simulink model "DrivingSimVR"  (Simulink 7.8)
settings: Solver=ode3  StartTime=0.0  StopTime=1000  FixedStep=0.05  RelTol=1e-3
PostLoadFcn:
  | load position
undefined symbols (not defined in the file or in its folder): serial
libraries: Conv_Lib x22, instrumentlib x2, vrlib x1
settings Model: Creator=CYJ  LastModifiedBy=rmchapin
settings DebuggingCC: FcnCallInpInsideContextMsg=Use local settings  StrictBusMsg=Warning

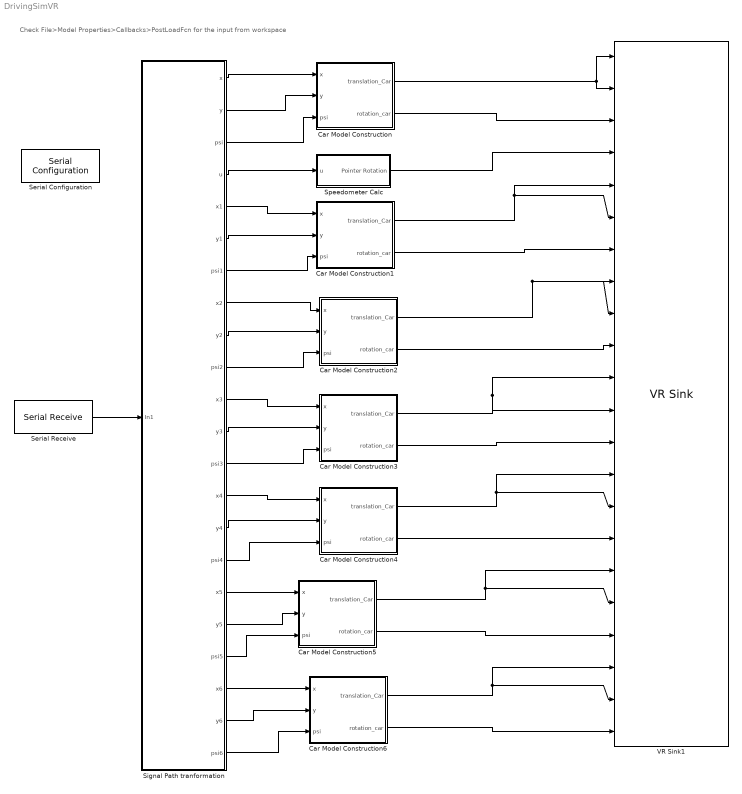
== system DrivingSimVR ==
  note: Check File>Model Properties>Callbacks>PostLoadFcn for the input from workspace
  Car Model Construction : Subsystem
  Car Model Construction1 : Subsystem
  Car Model Construction2 : Subsystem
  Car Model Construction3 : Subsystem
  Car Model Construction4 : Subsystem
  Car Model Construction5 : Subsystem
  Car Model Construction6 : Subsystem
  Serial Configuration : instrumentlib/Serial Configuration  Priority=-200000  ComPortMenu=COM1  ComPort=COM1  ObjConstructor=serial('COM1');  BaudRate=115200  DataBits=8  Parity=none  StopBits=1  FlowControl=none  Timeout=10  ByteOrder=BigEndian
  Serial Receive : instrumentlib/Serial Receive  ComPortMenu=COM1  ComPort=COM1  ObjConstructor=serial('COM1');  Header=s  Terminator=e  DataSize="[88   1]"  DataType=uint8  EnableBlockingMode=on  ActionDataUnavailable=Error  CustomValue=0  SampleTime=0.05
  Signal Path tranformation : Subsystem
  Speedometer Calc : Subsystem
  VR Sink1 : vrlib/VR Sink  SampleTime=0.05  ViewEnable=on  RemoteChange=off  RemoteView=off  FieldsWritten=Vehicle1.translation.3.1.1.double#Object1.translation.3.1.1.double#Car_Lotus1.rotation.4.1.1.double#Pointer.rotation.4.1.1.double#Vehicle2.translation.3.1.1.double#Object2.translation.3.1.1.double#Car_Lotus2.rotation.4.1.1.double#Vehicle3.translation.3.1.1.double#Object3.translation.3.1.1.double#Car_Lotus3.rotation.4.1.1.double#Vehicle4.translation.3.1.1.double#Object4.translation.3.1.1.double#Car_Lotus4.rotation.4.1.1.double#Vehicle5.translation.3.1.1.double#Object5.translation.3.1.1.double#Car_Lotus5.rotation.4.1.1.double#Vehicle6.translation.3.1.1.double#Object6.translation.3.1.1.double#Car_Lotus6.rotation.4.1.1.double#Vehicle7.translation.3.1.1.double#Object7.translation.3.1.1.double#Car_Lotus7.rotation.4.1.1.double  WorldFileName=path-11052012.wrl  AutoView=on  VideoDimensions=[]  AllowVariableSize=off
  wires:
  Serial Receive/1 -> Signal Path tranformation/1(In1)
  Signal Path tranformation/1(x) -> Car Model Construction/1(x)
  Signal Path tranformation/2(y) -> Car Model Construction/2(y)
  Signal Path tranformation/3(psi) -> Car Model Construction/3(psi)
  Signal Path tranformation/5(x1) -> Car Model Construction1/1(x)
  Signal Path tranformation/6(y1) -> Car Model Construction1/2(y)
  Signal Path tranformation/7(psi1) -> Car Model Construction1/3(psi)
  Signal Path tranformation/8(x2) -> Car Model Construction2/1(x)
  Signal Path tranformation/9(y2) -> Car Model Construction2/2(y)
  Signal Path tranformation/10(psi2) -> Car Model Construction2/3(psi)
  Signal Path tranformation/11(x3) -> Car Model Construction3/1(x)
  Signal Path tranformation/12(y3) -> Car Model Construction3/2(y)
  Signal Path tranformation/13(psi3) -> Car Model Construction3/3(psi)
  Signal Path tranformation/14(x4) -> Car Model Construction4/1(x)
  Signal Path tranformation/15(y4) -> Car Model Construction4/2(y)
  Signal Path tranformation/16(psi4) -> Car Model Construction4/3(psi)
  Signal Path tranformation/17(x5) -> Car Model Construction5/1(x)
  Signal Path tranformation/18(y5) -> Car Model Construction5/2(y)
  Signal Path tranformation/19(psi5) -> Car Model Construction5/3(psi)
  Signal Path tranformation/4(u) -> Speedometer Calc/1(u)
  Car Model Construction/1(translation_Car) -> VR Sink1/1, VR Sink1/2
  Car Model Construction1/1(translation_Car) -> VR Sink1/5, VR Sink1/6
  Car Model Construction/2(rotation_car) -> VR Sink1/3
  Speedometer Calc/1(Pointer Rotation) -> VR Sink1/4
  Car Model Construction1/2(rotation_car) -> VR Sink1/7
  Car Model Construction2/1(translation_Car) -> VR Sink1/8, VR Sink1/9
  Car Model Construction2/2(rotation_car) -> VR Sink1/10
  Car Model Construction3/1(translation_Car) -> VR Sink1/11, VR Sink1/12
  Car Model Construction3/2(rotation_car) -> VR Sink1/13
  Car Model Construction4/1(translation_Car) -> VR Sink1/14, VR Sink1/15
  Car Model Construction4/2(rotation_car) -> VR Sink1/16
  Car Model Construction5/1(translation_Car) -> VR Sink1/17, VR Sink1/18
  Car Model Construction5/2(rotation_car) -> VR Sink1/19
  Signal Path tranformation/20(x6) -> Car Model Construction6/1(x)
  Signal Path tranformation/21(y6) -> Car Model Construction6/2(y)
  Signal Path tranformation/22(psi6) -> Car Model Construction6/3(psi)
  Car Model Construction6/1(translation_Car) -> VR Sink1/20, VR Sink1/21
  Car Model Construction6/2(rotation_car) -> VR Sink1/22

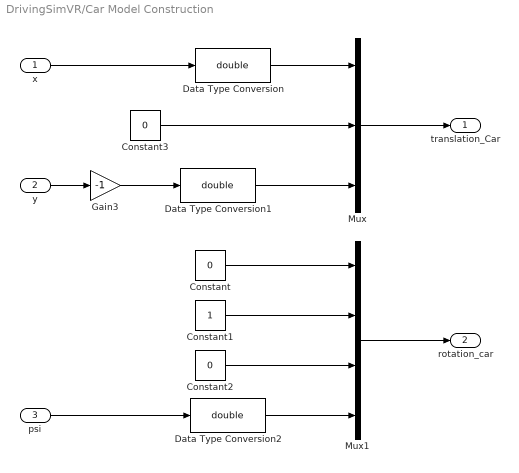
== system DrivingSimVR/Car Model Construction ==
  x : Inport
  y : Inport  Port=2
  psi : Inport  Port=3
  Constant : Constant  Value=0
  Constant1 : Constant
  Constant2 : Constant  Value=0
  Constant3 : Constant  Value=0
  Data Type Conversion : DataTypeConversion  OutDataTypeStr=double
  Data Type Conversion1 : DataTypeConversion  OutDataTypeStr=double
  Data Type Conversion2 : DataTypeConversion  OutDataTypeStr=double
  Gain3 : Gain  Gain=-1
  Mux : Mux  Inputs=3
  Mux1 : Mux
  translation_Car : Outport
  rotation_car : Outport  Port=2
  wires:
  Constant/1 -> Mux1/1
  Constant1/1 -> Mux1/2
  Constant2/1 -> Mux1/3
  Data Type Conversion2/1 -> Mux1/4
  y/1 -> Gain3/1
  psi/1 -> Data Type Conversion2/1
  Constant3/1 -> Mux/2
  Gain3/1 -> Data Type Conversion1/1
  x/1 -> Data Type Conversion/1
  Data Type Conversion1/1 -> Mux/3
  Data Type Conversion/1 -> Mux/1
  Mux/1 -> translation_Car/1
  Mux1/1 -> rotation_car/1

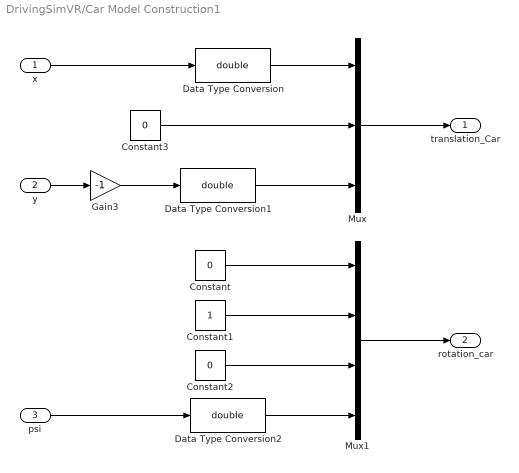
== system DrivingSimVR/Car Model Construction1 ==
  x : Inport
  y : Inport  Port=2
  psi : Inport  Port=3
  Constant : Constant  Value=0
  Constant1 : Constant
  Constant2 : Constant  Value=0
  Constant3 : Constant  Value=0
  Data Type Conversion : DataTypeConversion  OutDataTypeStr=double
  Data Type Conversion1 : DataTypeConversion  OutDataTypeStr=double
  Data Type Conversion2 : DataTypeConversion  OutDataTypeStr=double
  Gain3 : Gain  Gain=-1
  Mux : Mux  Inputs=3
  Mux1 : Mux
  translation_Car : Outport
  rotation_car : Outport  Port=2
  wires:
  Constant/1 -> Mux1/1
  Constant1/1 -> Mux1/2
  Constant2/1 -> Mux1/3
  Data Type Conversion2/1 -> Mux1/4
  y/1 -> Gain3/1
  psi/1 -> Data Type Conversion2/1
  Constant3/1 -> Mux/2
  Gain3/1 -> Data Type Conversion1/1
  x/1 -> Data Type Conversion/1
  Data Type Conversion1/1 -> Mux/3
  Data Type Conversion/1 -> Mux/1
  Mux/1 -> translation_Car/1
  Mux1/1 -> rotation_car/1

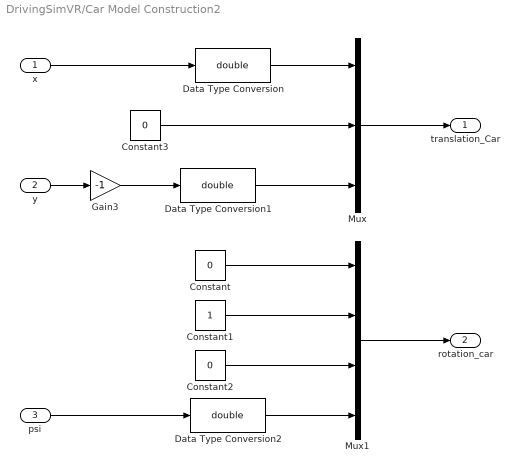
== system DrivingSimVR/Car Model Construction2 ==
  x : Inport
  y : Inport  Port=2
  psi : Inport  Port=3
  Constant : Constant  Value=0
  Constant1 : Constant
  Constant2 : Constant  Value=0
  Constant3 : Constant  Value=0
  Data Type Conversion : DataTypeConversion  OutDataTypeStr=double
  Data Type Conversion1 : DataTypeConversion  OutDataTypeStr=double
  Data Type Conversion2 : DataTypeConversion  OutDataTypeStr=double
  Gain3 : Gain  Gain=-1
  Mux : Mux  Inputs=3
  Mux1 : Mux
  translation_Car : Outport
  rotation_car : Outport  Port=2
  wires:
  Constant/1 -> Mux1/1
  Constant1/1 -> Mux1/2
  Constant2/1 -> Mux1/3
  Data Type Conversion2/1 -> Mux1/4
  y/1 -> Gain3/1
  psi/1 -> Data Type Conversion2/1
  Constant3/1 -> Mux/2
  Gain3/1 -> Data Type Conversion1/1
  x/1 -> Data Type Conversion/1
  Data Type Conversion1/1 -> Mux/3
  Data Type Conversion/1 -> Mux/1
  Mux/1 -> translation_Car/1
  Mux1/1 -> rotation_car/1

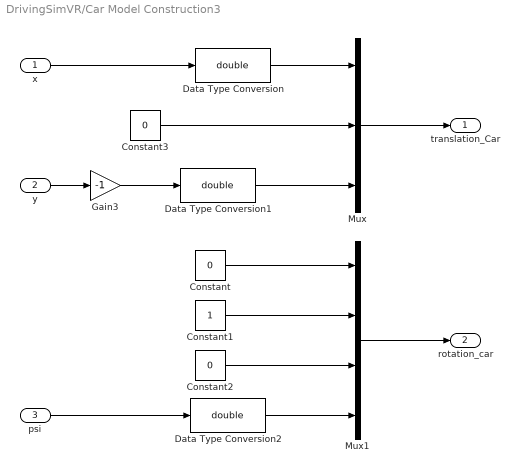
== system DrivingSimVR/Car Model Construction3 ==
  x : Inport
  y : Inport  Port=2
  psi : Inport  Port=3
  Constant : Constant  Value=0
  Constant1 : Constant
  Constant2 : Constant  Value=0
  Constant3 : Constant  Value=0
  Data Type Conversion : DataTypeConversion  OutDataTypeStr=double
  Data Type Conversion1 : DataTypeConversion  OutDataTypeStr=double
  Data Type Conversion2 : DataTypeConversion  OutDataTypeStr=double
  Gain3 : Gain  Gain=-1
  Mux : Mux  Inputs=3
  Mux1 : Mux
  translation_Car : Outport
  rotation_car : Outport  Port=2
  wires:
  Constant/1 -> Mux1/1
  Constant1/1 -> Mux1/2
  Constant2/1 -> Mux1/3
  Data Type Conversion2/1 -> Mux1/4
  y/1 -> Gain3/1
  psi/1 -> Data Type Conversion2/1
  Constant3/1 -> Mux/2
  Gain3/1 -> Data Type Conversion1/1
  x/1 -> Data Type Conversion/1
  Data Type Conversion1/1 -> Mux/3
  Data Type Conversion/1 -> Mux/1
  Mux/1 -> translation_Car/1
  Mux1/1 -> rotation_car/1

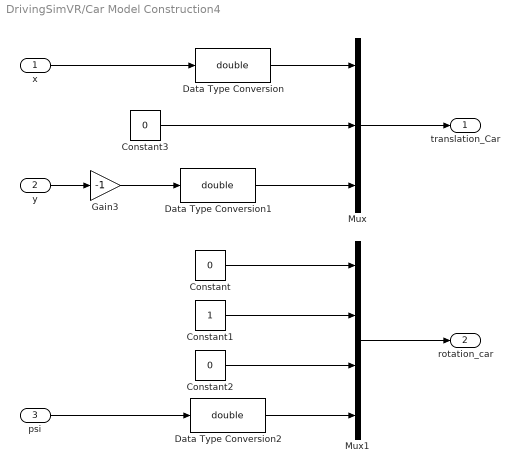
== system DrivingSimVR/Car Model Construction4 ==
  x : Inport
  y : Inport  Port=2
  psi : Inport  Port=3
  Constant : Constant  Value=0
  Constant1 : Constant
  Constant2 : Constant  Value=0
  Constant3 : Constant  Value=0
  Data Type Conversion : DataTypeConversion  OutDataTypeStr=double
  Data Type Conversion1 : DataTypeConversion  OutDataTypeStr=double
  Data Type Conversion2 : DataTypeConversion  OutDataTypeStr=double
  Gain3 : Gain  Gain=-1
  Mux : Mux  Inputs=3
  Mux1 : Mux
  translation_Car : Outport
  rotation_car : Outport  Port=2
  wires:
  Constant/1 -> Mux1/1
  Constant1/1 -> Mux1/2
  Constant2/1 -> Mux1/3
  Data Type Conversion2/1 -> Mux1/4
  y/1 -> Gain3/1
  psi/1 -> Data Type Conversion2/1
  Constant3/1 -> Mux/2
  Gain3/1 -> Data Type Conversion1/1
  x/1 -> Data Type Conversion/1
  Data Type Conversion1/1 -> Mux/3
  Data Type Conversion/1 -> Mux/1
  Mux/1 -> translation_Car/1
  Mux1/1 -> rotation_car/1

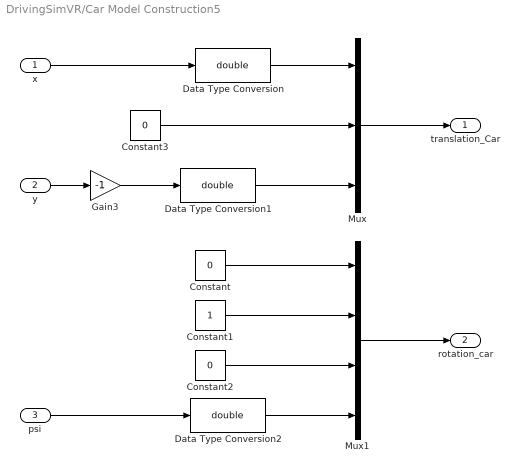
== system DrivingSimVR/Car Model Construction5 ==
  x : Inport
  y : Inport  Port=2
  psi : Inport  Port=3
  Constant : Constant  Value=0
  Constant1 : Constant
  Constant2 : Constant  Value=0
  Constant3 : Constant  Value=0
  Data Type Conversion : DataTypeConversion  OutDataTypeStr=double
  Data Type Conversion1 : DataTypeConversion  OutDataTypeStr=double
  Data Type Conversion2 : DataTypeConversion  OutDataTypeStr=double
  Gain3 : Gain  Gain=-1
  Mux : Mux  Inputs=3
  Mux1 : Mux
  translation_Car : Outport
  rotation_car : Outport  Port=2
  wires:
  Constant/1 -> Mux1/1
  Constant1/1 -> Mux1/2
  Constant2/1 -> Mux1/3
  Data Type Conversion2/1 -> Mux1/4
  y/1 -> Gain3/1
  psi/1 -> Data Type Conversion2/1
  Constant3/1 -> Mux/2
  Gain3/1 -> Data Type Conversion1/1
  x/1 -> Data Type Conversion/1
  Data Type Conversion1/1 -> Mux/3
  Data Type Conversion/1 -> Mux/1
  Mux/1 -> translation_Car/1
  Mux1/1 -> rotation_car/1

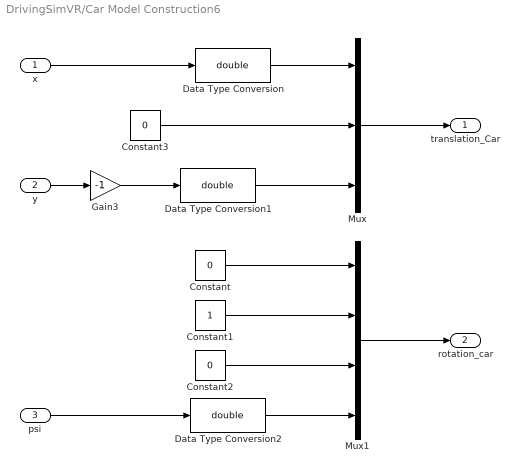
== system DrivingSimVR/Car Model Construction6 ==
  x : Inport
  y : Inport  Port=2
  psi : Inport  Port=3
  Constant : Constant  Value=0
  Constant1 : Constant
  Constant2 : Constant  Value=0
  Constant3 : Constant  Value=0
  Data Type Conversion : DataTypeConversion  OutDataTypeStr=double
  Data Type Conversion1 : DataTypeConversion  OutDataTypeStr=double
  Data Type Conversion2 : DataTypeConversion  OutDataTypeStr=double
  Gain3 : Gain  Gain=-1
  Mux : Mux  Inputs=3
  Mux1 : Mux
  translation_Car : Outport
  rotation_car : Outport  Port=2
  wires:
  Constant/1 -> Mux1/1
  Constant1/1 -> Mux1/2
  Constant2/1 -> Mux1/3
  Data Type Conversion2/1 -> Mux1/4
  y/1 -> Gain3/1
  psi/1 -> Data Type Conversion2/1
  Constant3/1 -> Mux/2
  Gain3/1 -> Data Type Conversion1/1
  x/1 -> Data Type Conversion/1
  Data Type Conversion1/1 -> Mux/3
  Data Type Conversion/1 -> Mux/1
  Mux/1 -> translation_Car/1
  Mux1/1 -> rotation_car/1

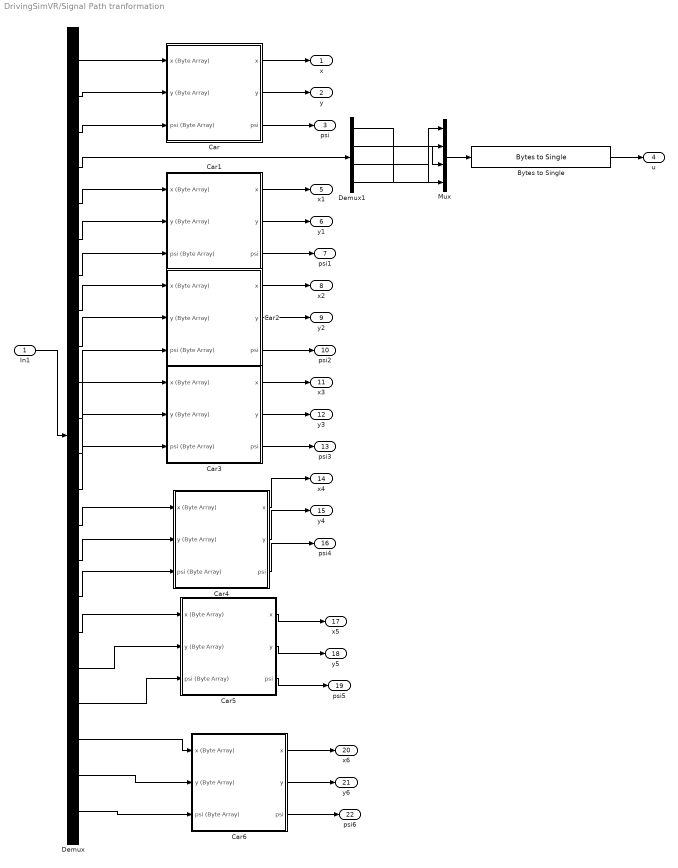
== system DrivingSimVR/Signal Path tranformation ==
  In1 : Inport
  Bytes to Single : Conv_Lib/Bytes to Single
  Car : Subsystem
  Car1 : Subsystem
  Car2 : Subsystem
  Car3 : Subsystem
  Car4 : Subsystem
  Car5 : Subsystem
  Car6 : Subsystem
  Demux : Demux  Outputs=22
  Demux1 : Demux
  Mux : Mux
  x : Outport
  y : Outport  Port=2
  psi : Outport  Port=3
  u : Outport  Port=4
  x1 : Outport  Port=5
  y1 : Outport  Port=6
  psi1 : Outport  Port=7
  x2 : Outport  Port=8
  y2 : Outport  Port=9
  psi2 : Outport  Port=10
  x3 : Outport  Port=11
  y3 : Outport  Port=12
  psi3 : Outport  Port=13
  x4 : Outport  Port=14
  y4 : Outport  Port=15
  psi4 : Outport  Port=16
  x5 : Outport  Port=17
  y5 : Outport  Port=18
  psi5 : Outport  Port=19
  x6 : Outport  Port=20
  y6 : Outport  Port=21
  psi6 : Outport  Port=22
  wires:
  In1/1 -> Demux/1
  Car/1(x) -> x/1
  Car/2(y) -> y/1
  Car/3(psi) -> psi/1
  Demux/1 -> Car/1(x (Byte Array))
  Demux/2 -> Car/2(y (Byte Array))
  Demux/3 -> Car/3(psi (Byte Array))
  Bytes to Single/1 -> u/1
  Car1/1(x) -> x1/1
  Car1/2(y) -> y1/1
  Car1/3(psi) -> psi1/1
  Car2/1(x) -> x2/1
  Car2/2(y) -> y2/1
  Car2/3(psi) -> psi2/1
  Car3/1(x) -> x3/1
  Car3/2(y) -> y3/1
  Car3/3(psi) -> psi3/1
  Car4/1(x) -> x4/1
  Car4/2(y) -> y4/1
  Car4/3(psi) -> psi4/1
  Car5/1(x) -> x5/1
  Car5/2(y) -> y5/1
  Car5/3(psi) -> psi5/1
  Demux/5 -> Car1/1(x (Byte Array))
  Demux/6 -> Car1/2(y (Byte Array))
  Demux/7 -> Car1/3(psi (Byte Array))
  Demux/8 -> Car2/1(x (Byte Array))
  Demux/9 -> Car2/2(y (Byte Array))
  Demux/10 -> Car2/3(psi (Byte Array))
  Demux/11 -> Car3/1(x (Byte Array))
  Demux/12 -> Car3/2(y (Byte Array))
  Demux/13 -> Car3/3(psi (Byte Array))
  Demux/14 -> Car4/1(x (Byte Array))
  Demux/15 -> Car4/2(y (Byte Array))
  Demux/16 -> Car4/3(psi (Byte Array))
  Mux/1 -> Bytes to Single/1
  Demux1/1 -> Mux/4
  Demux1/2 -> Mux/3
  Demux1/3 -> Mux/2
  Demux1/4 -> Mux/1
  Demux/4 -> Demux1/1
  Car6/1(x) -> x6/1
  Car6/2(y) -> y6/1
  Car6/3(psi) -> psi6/1
  Demux/17 -> Car5/1(x (Byte Array))
  Demux/18 -> Car5/2(y (Byte Array))
  Demux/19 -> Car5/3(psi (Byte Array))
  Demux/20 -> Car6/1(x (Byte Array))
  Demux/21 -> Car6/2(y (Byte Array))
  Demux/22 -> Car6/3(psi (Byte Array))

== system DrivingSimVR/Speedometer Calc ==
  u : Inport
  Constant : Constant  Value=0
  Constant1 : Constant  Value=0
  Constant2 : Constant
  Data Type Conversion2 : DataTypeConversion  OutDataTypeStr=double
  Gain : Gain  Gain=-(pi)/55
  Mux1 : Mux
  Pointer Rotation : Outport
  wires:
  Constant/1 -> Mux1/1
  Constant1/1 -> Mux1/2
  Constant2/1 -> Mux1/3
  Data Type Conversion2/1 -> Mux1/4
  Gain/1 -> Data Type Conversion2/1
  u/1 -> Gain/1
  Mux1/1 -> Pointer Rotation/1

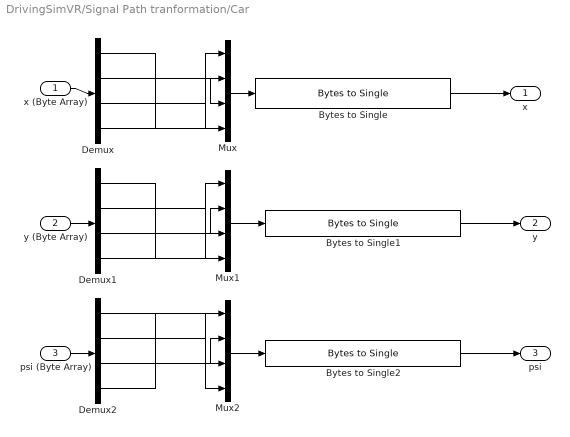
== system DrivingSimVR/Signal Path tranformation/Car ==
  x (Byte Array) : Inport
  y (Byte Array) : Inport  Port=2
  psi (Byte Array) : Inport  Port=3
  Bytes to Single : Conv_Lib/Bytes to Single
  Bytes to Single1 : Conv_Lib/Bytes to Single
  Bytes to Single2 : Conv_Lib/Bytes to Single
  Demux : Demux
  Demux1 : Demux
  Demux2 : Demux
  Mux : Mux
  Mux1 : Mux
  Mux2 : Mux
  x : Outport
  y : Outport  Port=2
  psi : Outport  Port=3
  wires:
  Bytes to Single/1 -> x/1
  Bytes to Single1/1 -> y/1
  Bytes to Single2/1 -> psi/1
  x (Byte Array)/1 -> Demux/1
  y (Byte Array)/1 -> Demux1/1
  psi (Byte Array)/1 -> Demux2/1
  Mux/1 -> Bytes to Single/1
  Mux1/1 -> Bytes to Single1/1
  Mux2/1 -> Bytes to Single2/1
  Demux/1 -> Mux/4
  Demux/2 -> Mux/3
  Demux/3 -> Mux/2
  Demux/4 -> Mux/1
  Demux1/1 -> Mux1/4
  Demux1/4 -> Mux1/1
  Demux1/3 -> Mux1/2
  Demux1/2 -> Mux1/3
  Demux2/4 -> Mux2/1
  Demux2/1 -> Mux2/4
  Demux2/3 -> Mux2/2
  Demux2/2 -> Mux2/3

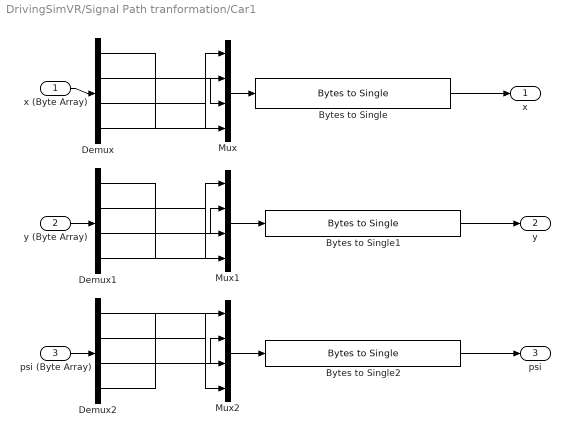
== system DrivingSimVR/Signal Path tranformation/Car1 ==
  x (Byte Array) : Inport
  y (Byte Array) : Inport  Port=2
  psi (Byte Array) : Inport  Port=3
  Bytes to Single : Conv_Lib/Bytes to Single
  Bytes to Single1 : Conv_Lib/Bytes to Single
  Bytes to Single2 : Conv_Lib/Bytes to Single
  Demux : Demux
  Demux1 : Demux
  Demux2 : Demux
  Mux : Mux
  Mux1 : Mux
  Mux2 : Mux
  x : Outport
  y : Outport  Port=2
  psi : Outport  Port=3
  wires:
  Bytes to Single/1 -> x/1
  Bytes to Single1/1 -> y/1
  Bytes to Single2/1 -> psi/1
  x (Byte Array)/1 -> Demux/1
  y (Byte Array)/1 -> Demux1/1
  psi (Byte Array)/1 -> Demux2/1
  Mux/1 -> Bytes to Single/1
  Mux1/1 -> Bytes to Single1/1
  Mux2/1 -> Bytes to Single2/1
  Demux/1 -> Mux/4
  Demux/2 -> Mux/3
  Demux/3 -> Mux/2
  Demux/4 -> Mux/1
  Demux1/1 -> Mux1/4
  Demux1/4 -> Mux1/1
  Demux1/3 -> Mux1/2
  Demux1/2 -> Mux1/3
  Demux2/4 -> Mux2/1
  Demux2/1 -> Mux2/4
  Demux2/3 -> Mux2/2
  Demux2/2 -> Mux2/3

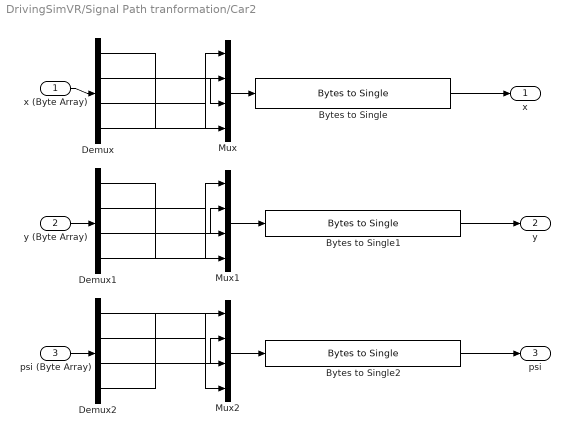
== system DrivingSimVR/Signal Path tranformation/Car2 ==
  x (Byte Array) : Inport
  y (Byte Array) : Inport  Port=2
  psi (Byte Array) : Inport  Port=3
  Bytes to Single : Conv_Lib/Bytes to Single
  Bytes to Single1 : Conv_Lib/Bytes to Single
  Bytes to Single2 : Conv_Lib/Bytes to Single
  Demux : Demux
  Demux1 : Demux
  Demux2 : Demux
  Mux : Mux
  Mux1 : Mux
  Mux2 : Mux
  x : Outport
  y : Outport  Port=2
  psi : Outport  Port=3
  wires:
  Bytes to Single/1 -> x/1
  Bytes to Single1/1 -> y/1
  Bytes to Single2/1 -> psi/1
  x (Byte Array)/1 -> Demux/1
  y (Byte Array)/1 -> Demux1/1
  psi (Byte Array)/1 -> Demux2/1
  Mux/1 -> Bytes to Single/1
  Mux1/1 -> Bytes to Single1/1
  Mux2/1 -> Bytes to Single2/1
  Demux/1 -> Mux/4
  Demux/2 -> Mux/3
  Demux/3 -> Mux/2
  Demux/4 -> Mux/1
  Demux1/1 -> Mux1/4
  Demux1/4 -> Mux1/1
  Demux1/3 -> Mux1/2
  Demux1/2 -> Mux1/3
  Demux2/4 -> Mux2/1
  Demux2/1 -> Mux2/4
  Demux2/3 -> Mux2/2
  Demux2/2 -> Mux2/3

== system DrivingSimVR/Signal Path tranformation/Car3 ==
  x (Byte Array) : Inport
  y (Byte Array) : Inport  Port=2
  psi (Byte Array) : Inport  Port=3
  Bytes to Single : Conv_Lib/Bytes to Single
  Bytes to Single1 : Conv_Lib/Bytes to Single
  Bytes to Single2 : Conv_Lib/Bytes to Single
  Demux : Demux
  Demux1 : Demux
  Demux2 : Demux
  Mux : Mux
  Mux1 : Mux
  Mux2 : Mux
  x : Outport
  y : Outport  Port=2
  psi : Outport  Port=3
  wires:
  Bytes to Single/1 -> x/1
  Bytes to Single1/1 -> y/1
  Bytes to Single2/1 -> psi/1
  x (Byte Array)/1 -> Demux/1
  y (Byte Array)/1 -> Demux1/1
  psi (Byte Array)/1 -> Demux2/1
  Mux/1 -> Bytes to Single/1
  Mux1/1 -> Bytes to Single1/1
  Mux2/1 -> Bytes to Single2/1
  Demux/1 -> Mux/4
  Demux/2 -> Mux/3
  Demux/3 -> Mux/2
  Demux/4 -> Mux/1
  Demux1/1 -> Mux1/4
  Demux1/4 -> Mux1/1
  Demux1/3 -> Mux1/2
  Demux1/2 -> Mux1/3
  Demux2/4 -> Mux2/1
  Demux2/1 -> Mux2/4
  Demux2/3 -> Mux2/2
  Demux2/2 -> Mux2/3

== system DrivingSimVR/Signal Path tranformation/Car4 ==
  x (Byte Array) : Inport
  y (Byte Array) : Inport  Port=2
  psi (Byte Array) : Inport  Port=3
  Bytes to Single : Conv_Lib/Bytes to Single
  Bytes to Single1 : Conv_Lib/Bytes to Single
  Bytes to Single2 : Conv_Lib/Bytes to Single
  Demux : Demux
  Demux1 : Demux
  Demux2 : Demux
  Mux : Mux
  Mux1 : Mux
  Mux2 : Mux
  x : Outport
  y : Outport  Port=2
  psi : Outport  Port=3
  wires:
  Bytes to Single/1 -> x/1
  Bytes to Single1/1 -> y/1
  Bytes to Single2/1 -> psi/1
  x (Byte Array)/1 -> Demux/1
  y (Byte Array)/1 -> Demux1/1
  psi (Byte Array)/1 -> Demux2/1
  Mux/1 -> Bytes to Single/1
  Mux1/1 -> Bytes to Single1/1
  Mux2/1 -> Bytes to Single2/1
  Demux/1 -> Mux/4
  Demux/2 -> Mux/3
  Demux/3 -> Mux/2
  Demux/4 -> Mux/1
  Demux1/1 -> Mux1/4
  Demux1/4 -> Mux1/1
  Demux1/3 -> Mux1/2
  Demux1/2 -> Mux1/3
  Demux2/4 -> Mux2/1
  Demux2/1 -> Mux2/4
  Demux2/3 -> Mux2/2
  Demux2/2 -> Mux2/3

== system DrivingSimVR/Signal Path tranformation/Car5 ==
  x (Byte Array) : Inport
  y (Byte Array) : Inport  Port=2
  psi (Byte Array) : Inport  Port=3
  Bytes to Single : Conv_Lib/Bytes to Single
  Bytes to Single1 : Conv_Lib/Bytes to Single
  Bytes to Single2 : Conv_Lib/Bytes to Single
  Demux : Demux
  Demux1 : Demux
  Demux2 : Demux
  Mux : Mux
  Mux1 : Mux
  Mux2 : Mux
  x : Outport
  y : Outport  Port=2
  psi : Outport  Port=3
  wires:
  Bytes to Single/1 -> x/1
  Bytes to Single1/1 -> y/1
  Bytes to Single2/1 -> psi/1
  x (Byte Array)/1 -> Demux/1
  y (Byte Array)/1 -> Demux1/1
  psi (Byte Array)/1 -> Demux2/1
  Mux/1 -> Bytes to Single/1
  Mux1/1 -> Bytes to Single1/1
  Mux2/1 -> Bytes to Single2/1
  Demux/1 -> Mux/4
  Demux/2 -> Mux/3
  Demux/3 -> Mux/2
  Demux/4 -> Mux/1
  Demux1/1 -> Mux1/4
  Demux1/4 -> Mux1/1
  Demux1/3 -> Mux1/2
  Demux1/2 -> Mux1/3
  Demux2/4 -> Mux2/1
  Demux2/1 -> Mux2/4
  Demux2/3 -> Mux2/2
  Demux2/2 -> Mux2/3

== system DrivingSimVR/Signal Path tranformation/Car6 ==
  x (Byte Array) : Inport
  y (Byte Array) : Inport  Port=2
  psi (Byte Array) : Inport  Port=3
  Bytes to Single : Conv_Lib/Bytes to Single
  Bytes to Single1 : Conv_Lib/Bytes to Single
  Bytes to Single2 : Conv_Lib/Bytes to Single
  Demux : Demux
  Demux1 : Demux
  Demux2 : Demux
  Mux : Mux
  Mux1 : Mux
  Mux2 : Mux
  x : Outport
  y : Outport  Port=2
  psi : Outport  Port=3
  wires:
  Bytes to Single/1 -> x/1
  Bytes to Single1/1 -> y/1
  Bytes to Single2/1 -> psi/1
  x (Byte Array)/1 -> Demux/1
  y (Byte Array)/1 -> Demux1/1
  psi (Byte Array)/1 -> Demux2/1
  Mux/1 -> Bytes to Single/1
  Mux1/1 -> Bytes to Single1/1
  Mux2/1 -> Bytes to Single2/1
  Demux/1 -> Mux/4
  Demux/2 -> Mux/3
  Demux/3 -> Mux/2
  Demux/4 -> Mux/1
  Demux1/1 -> Mux1/4
  Demux1/4 -> Mux1/1
  Demux1/3 -> Mux1/2
  Demux1/2 -> Mux1/3
  Demux2/4 -> Mux2/1
  Demux2/1 -> Mux2/4
  Demux2/3 -> Mux2/2
  Demux2/2 -> Mux2/3
